simulink model "fixed_model"  (R2024a)
settings: Solver=VariableStepAuto  StartTime=0.0  StopTime=1  RelTol=1e-3
undefined symbols (not defined in the file or in its folder): Radix, SAMPLING_FREQ, signal_1
libraries: dspstat3 x2, dspxfrm3 x1, dspsrcs4 x1, simulink x1
settings Model: SimulationMode=accelerator  Creator=Jan Rosa  LastModifiedBy=Jan Rosa
settings HardwareCC: ProdBitPerPointer=32  ProdBitPerSizeT=32  ProdBitPerPtrDiffT=32  ProdLargestAtomicFloat=None  ProdIntDivRoundTo=Undefined  ProdEndianess=Unspecified  ProdWordSize=32  ProdHWDeviceType=ASIC/FPGA->ASIC/FPGA  TargetBitPerPointer=64  TargetBitPerSizeT=64  TargetBitPerPtrDiffT=64  TargetLongLongMode=on  TargetIntDivRoundTo=Zero  TargetEndianess=LittleEndian  TargetWordSize=64  TargetHWDeviceType=Custom Processor->MATLAB Host Computer  ProdEqTarget=off

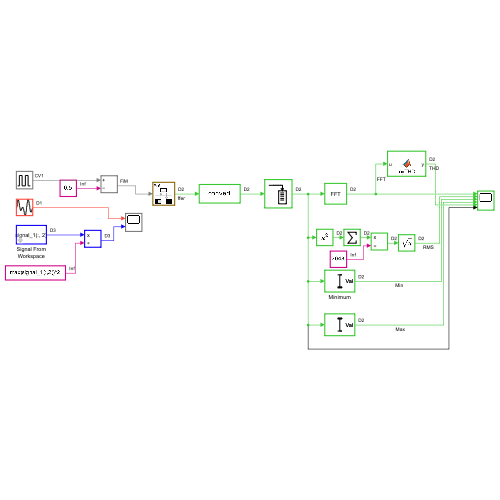
[thumbnail: Simulink's stored preview of the top-level diagram]
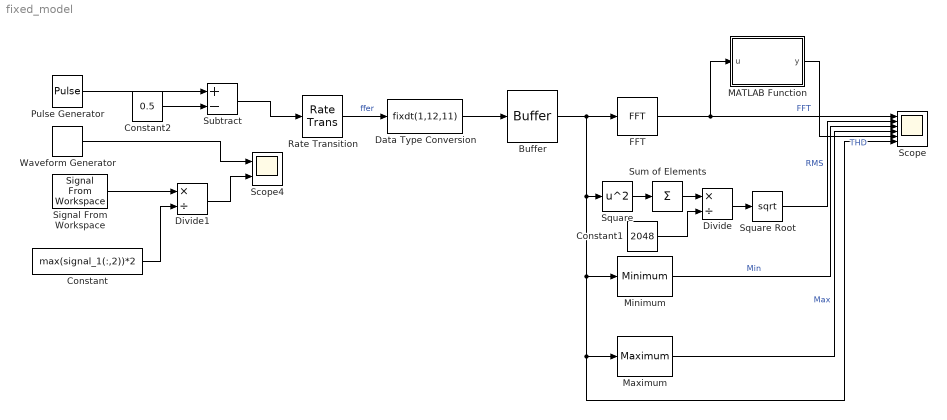
== system fixed_model ==
  Buffer : Buffer  N=2048  V=2047  OutputFrames=off
  Constant : Constant  Value=max(signal_1(:,2))*2
  Constant1 : Constant  Value=2048  OutDataTypeStr=fixdt(0,12,0)
  Constant2 : Constant  Value=0.5
  Data Type Conversion : DataTypeConversion  OutDataTypeStr=fixdt(1,12,11)  SaturateOnIntegerOverflow=off  RndMeth=Floor
  Divide : Product  Inputs=*/
  Divide1 : Product  Inputs=*/
  FFT : dspxfrm3/FFT  FFTImplementation=Radix-2  CompMethod=Table lookup  TableOpt=NEW  TableOptActive=Speed  BitRevOrder=off  Normalize=on  InheritFFTLength=on  FFTLength=64  WrapInput=on  roundingMode=Ceiling  overflowMode=on  firstCoeffDataTypeStr=Inherit: Same word length as input  firstCoeffLastDataTypeStr=Inherit: Same word length as input  prodOutputMode=Binary point scaling  prodOutputWordLength=32  prodOutputFracLength=12  prodOutputDataTypeStr=fixdt(1,32,12)  prodOutputLastDataTypeStr=fixdt(1,32,12)  accumMode=Binary point scaling  accumWordLength=32  accumFracLength=12  accumDataTypeStr=fixdt(1,32,12)  accumLastDataTypeStr=fixdt(1,32,12)  outputMin=[]  outputMax=[]
      settings: LockScale=on
  MATLAB Function : MATLAB Function  TreatAsAtomicUnit=on
  Maximum : dspstat3/Maximum  operation=maximum  fcn=Value  indexBase=One  operateOver=Each column  Dimension=1  InputProcessing=Columns as channels (frame based)  reset=None  roiEnable=off  roiType=Rectangles  roiPortion=Entire ROI  roiOutput=Individual statistics for each ROI  roiFlag=off  roundingMode=Floor  overflowMode=off  prodOutputMode=Binary point scaling  prodOutputWordLength=13  prodOutputFracLength=12  prodOutputDataTypeStr=fixdt([],13,12)  prodOutputLastDataTypeStr=fixdt([],13,12)  accumDataTypeStr=Inherit: Same as product output  accumLastDataTypeStr=Inherit: Same as product output
      settings: LockScale=on
  Minimum : dspstat3/Minimum  operation=minimum  fcn=Value  indexBase=One  operateOver=Entire input  Dimension=1  InputProcessing=Columns as channels (frame based)  reset=None  roiEnable=off  roiType=Rectangles  roiPortion=Entire ROI  roiOutput=Individual statistics for each ROI  roiFlag=off  roundingMode=Floor  overflowMode=off  prodOutputMode=Binary point scaling  prodOutputWordLength=13  prodOutputFracLength=12  prodOutputDataTypeStr=fixdt([],13,12)  prodOutputLastDataTypeStr=fixdt([],13,12)  accumDataTypeStr=Inherit: Same as product output  accumLastDataTypeStr=Inherit: Same as product output
      settings: LibrarySourceBlock=dsphdlsupportstat/Minimum  LockScale=on
  Pulse Generator : DiscretePulseGenerator  PulseType=Time based  Amplitude=0.999  Period=1/50  PulseWidth=50
  Rate Transition : RateTransition  Deterministic=off  OutPortSampleTime=1/SAMPLING_FREQ
  Scope : Scope  NumInputPorts=6
  Scope4 : Scope  NumInputPorts=2
  Signal From Workspace : dspsrcs4/Signal From Workspace  X=signal_1(:, 2)  Ts=signal_1(2, 1)  nsamps=1  OutputAfterFinalValue=Cyclic repetition  ignoreOrWarnInputAndFrameLengths=off  OutputFrames=off
  Square : Math  Operator=square
  Square Root : Sqrt
  Subtract : Sum  Inputs=+-
  Sum of Elements : Sum  Inputs=+  InputSameDT=on  SaturateOnIntegerOverflow=on
  Waveform Generator : simulink/Sources/Waveform Generator  OutMin=[]  OutMax=[]  OutDataTypeStr=double  SelectedSignal=1  Signals=0.99*sin(0.5, 50*2*pi, 0)  BlockNames=MultiportSwitch_c7ceefe4d1e8441  SampleTime=1/(SAMPLING_FREQ*2)
  wires:
  Rate Transition/1 -> Data Type Conversion/1  "ffer"
  Maximum/1 -> Scope/4  "Max"
  Data Type Conversion/1 -> Buffer/1
  FFT/1 -> MATLAB Function/1(u), Scope/1  "FFT"
  Minimum/1 -> Scope/3  "Min"
  Buffer/1 -> FFT/1, Scope/6, Maximum/1, Minimum/1, Square/1
  Divide/1 -> Square Root/1
  Sum of Elements/1 -> Divide/1
  Constant1/1 -> Divide/2
  Square/1 -> Sum of Elements/1
  Square Root/1 -> Scope/2  "RMS"
  Signal From Workspace/1 -> Divide1/1
  Constant/1 -> Divide1/2
  Waveform Generator/1 -> Scope4/1
  MATLAB Function/1(y) -> Scope/5  "THD"
  Divide1/1 -> Scope4/2
  Pulse Generator/1 -> Subtract/1
  Constant2/1 -> Subtract/2
  Subtract/1 -> Rate Transition/1

== matlab function fixed_model/MATLAB Function ==
  data: u input; y output
function y = myTHD(u)

    main_frequency_index = 9;
    u_re = abs(u);
    halfway_index = floor(length(u_re) / 2); % Calculate the halfway point
    
y = sqrt(sum(u_re(main_frequency_index+1:halfway_index).^2))/u_re(main_frequency_index);
